simulink model "RealCar_pedestrian"  (R2024b)
settings: Solver=VariableStepAuto  StartTime=0.0  StopTime=inf  RelTol=1e-3
values from neighbouring files (symbols this model uses):
  C = [1 0 0 0; 0 1 0 0]    [Car_test_UDP.m]    (also in Final_Code_GPS.m; Final_Code_plotting_reset_kalman.m; KalmanFilter.m)
libraries: sim3dautolib x3, sim3dlib x1
settings Model: Creator=ritvi  LastModifiedBy=ritvi

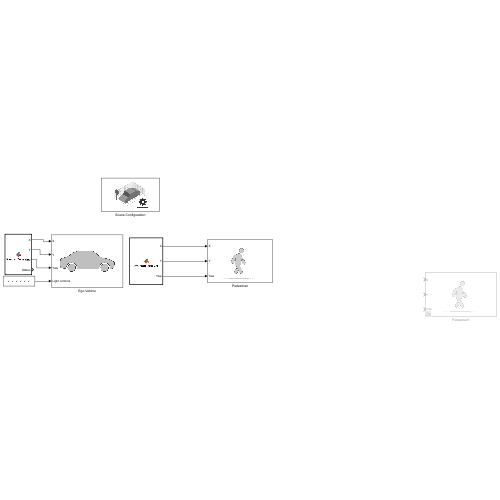
[thumbnail: Simulink's stored preview of the top-level diagram]
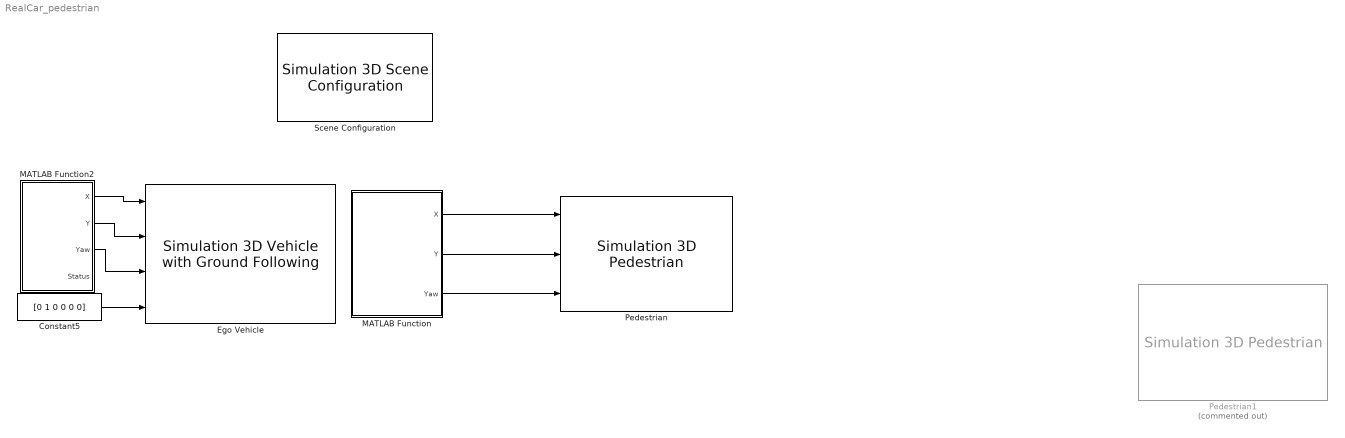
== system RealCar_pedestrian ==
  Constant5 : Constant  Value=[0 1 0 0 0 0]
  Ego Vehicle : sim3dautolib/Simulation 3D Vehicle with Ground Following  Priority=-1  PassVehMesh=Hatchback  MeshPath=/MathWorksSimulation/Vehicles/Muscle/Meshes/SK_MuscleCar.SK_MuscleCar  TrackWidth=1.9  WheelBase=3  WheelRadius=0.35  VehColor=Red  InitialPos=[15, 15, 0]  InitialRot=[0, 0, 90]  ActorName=SimulinkVehicle2  SampleTime=-1  ActorType=SimulinkVehicle  ID=2  aMode=3  ActorTag=SimulinkVehicle2  CoordinateScheme=ISO  VehLightsControl=on  HeadlightColor=[ 1, 1, 1 ]  HighBeamIntensity=100000  LowBeamIntensity=60000  HighBeamConeAngle=70  LowBeamConeAngle=70  LeftHeadlightOrientation=[ 0, 0 ]  RightHeadlightOrientation=[ 0, 0 ]  BrakelightIntensity=500  ReverselightIntensity=500  SignallightIntensity=500  SignallightPeriod=1  SignalPulseWidth=50  TransformOutportEnabled=off
      settings: LibrarySourceBlock=drivingsim3d/Simulation 3D Vehicle with Ground Following
  MATLAB Function : MATLAB Function  TreatAsAtomicUnit=on
  MATLAB Function2 : MATLAB Function  TreatAsAtomicUnit=on
  Pedestrian : sim3dautolib/Simulation 3D Pedestrian  Priority=-1  PedestrianType=Female 1  Scale=[1, 1, 1]  InitialPos=[35, 10, 0]  InitialYaw=0  ActorName=SimulinkPedestrian2  SampleTime=-1  ActorType=SimulinkPedestrian  ActorTag=SimulinkPedestrian2  ID=2  aMode=3  CoordinateScheme=ISO  TransformOutportEnabled=off
      settings: LibrarySourceBlock=drivingsim3d/Simulation 3D Pedestrian
  Pedestrian1 : sim3dautolib/Simulation 3D Pedestrian  Priority=-1  Commented=on  PedestrianType=Female 1  Scale=[1, 1, 1]  InitialPos=[0, 0, 0]  InitialYaw=0  ActorName=SimulinkPedestrian3  SampleTime=-1  ActorType=SimulinkPedestrian  ActorTag=SimulinkPedestrian3  ID=3  aMode=3  CoordinateScheme=ISO  TransformOutportEnabled=off
      settings: LibrarySourceBlock=drivingsim3d/Simulation 3D Pedestrian
  Scene Configuration : sim3dlib/Simulation 3D Scene Configuration  Priority=0  ProjectFormat=Unreal Editor  SceneDesc=Large parking lot  ProjectName=C:\Program Files\MATLAB\R2024b\toolbox\shared\sim3d_projects\automotive_project_windows\UE\WindowsNoEditor\VehicleSimulation.exe  ScenePath=/Game/Maps/HwStrght  UEProjPath=C:\Local\AutoVrtlEnv\AutoVrtlEnv.uproject  EnableOpenDRIVE=off  vehTagList={'Custom';'Scene Origin';'SimulinkVehicle2'}  vehTag=SimulinkVehicle2  FreeCameraInitialTranslation=[0, 0, 0]  FreeCameraDefaultInitialTranslation=[-6, 0, 2]  FreeCameraInitialRotation=[0, 0, 0]  FreeCameraDefaultInitialRotation=[0, -15, 0]  OpVisEn=off  Ts=0.05  EnableWindow=on  EnableRemoteAccess=off  EnableWeather=off  SunAzimuth=183.600  SunAltitude=0.0  EnableGeospatialSun=off  Latitude=0  Longitude=0  Date=2023-01-01  Time=10:30:00  GeoTimeZone=-5.0  SunDaylightSaving=off  wind=1  clouds=50.0  EnableVolumetricClouds=off  CloudCoverage=0  CloudAltitude=6  fog=0.0  rain=18.0  RaindropsEffect=off  SnowDensity=0  EnableGeospatial=off  UseTrueOrigin=off  OriginHeight=200  OriginLatitude=40.744652  OriginLongitude=-73.988864  MapStyle=Aerial  AdditionalAssetIDs=[]  UseAdvancedSunSky=off  SolarTime=11  TimeZone=-5  Day=21  Month=9  Year=2022  UseDaylightSavingTime=on  DSTStartDay=10  DSTStartMonth=3  DSTEndDay=3  DSTEndMonth=11  DSTSwitchHour=2  sensorTag=MainCamera2  sensorId=2  sensorName=MainCamera2  mountLoc=Origin  offsetFlag=off  tmountOffset=[0, 0, 0]  rmountOffset=[0, 0, 0]  HorizontalResolution=1280  VerticalResolution=720  HorizontalFOV=60  mountPoint=[0 0 0]  mountOrientation=[0 0 0]  aMode=3  ID=2  GeoTrigger=Inactive
      settings: LibrarySourceBlock=drivingsim3d/Simulation 3D Scene Configuration
  wires:
  Constant5/1 -> Ego Vehicle/4
  MATLAB Function2/1(X) -> Ego Vehicle/1
  MATLAB Function/3(Yaw) -> Pedestrian/3
  MATLAB Function/2(Y) -> Pedestrian/2
  MATLAB Function/1(X) -> Pedestrian/1
  MATLAB Function2/2(Y) -> Ego Vehicle/2
  MATLAB Function2/3(Yaw) -> Ego Vehicle/3

== matlab function RealCar_pedestrian/MATLAB Function ==
  data: X output; Y output; Yaw output
function [X, Y, Yaw] = livePedReceiver()
%#codegen
coder.extrinsic('evalin', 'exist');

% 1. Set safe defaults to MATCH the 15m offset!
X = 15.0;
Y = 15.0;
Yaw = 0.0;

% 2. Check the workspace for the newest target location
if evalin('base', 'exist(''Ped_X'', ''var'')')
    
    % Pull the live pedestrian data directly from the workspace
    X   = evalin('base', 'Ped_X');
    Y   = evalin('base', 'Ped_Y');
    Yaw = evalin('base', 'Ped_Yaw');
    
end

== matlab function RealCar_pedestrian/MATLAB Function2 ==
  data: X output; Y output; Yaw output; Status output
function [X, Y, Yaw, Status] = liveCarReceiver()
%#codegen
coder.extrinsic('evalin', 'exist');

% 1. Set safe defaults to MATCH the 15m offset!
X = 15.0;
Y = 15.0;
Yaw = 0.0;
Status = 0.0;

% 2. Check the workspace for the newest target location
if evalin('base', 'exist(''Car_X'', ''var'')')
    
    % Pull the live car data directly from the workspace
    X      = evalin('base', 'Car_X');
    Y      = evalin('base', 'Car_Y');
    Yaw    = evalin('base', 'Car_Yaw');
    Status = evalin('base', 'Car_Status');
    
end
